simulink model "AerodynamicMoment"  (R2023b)
settings: Solver=VariableStepAuto  StartTime=0.0  StopTime=Tfinal  RelTol=1e-3
model workspace (MAT data in the model file):
  areas = [26.28; 12; 3; 7.5; 17.1; 53.96; 53.96; 4.5; 26.28; 20.1]
  centroids = [4.30109589041  0  1.69726027397; 8.04  1.25  2.4; 7.44  1.25  4.8; 0  1.25  1.5; 3.42  1.25  3; 4.02  9.6  2.3; 4.02  9.6  2.3; 6.84  1.25  3.9; 4.30109589041  0  1.69726027397; 4.02  1.25  0]
  normalVectors = [0  -1  0; 1  0  0; 0  0  1; -1  0  0; 0  0  1; 0  0  1; 0  0  -1; -1  0  0; 0  1  0; 0  0  -1]
  rcm = [4.05894270882 1.95833333333 1.80412649485]
  sequence = "313"
  u0 = [2.10277093747; 1.71391332546; 1.66166340364]
values from neighbouring files (symbols this model uses):
  A_ptob = [0.00452111179393  0.994865050863  -0.101109297888; -0.99864921572  -0.000741813086313  -0.051953764597; -0.0517619888586  0.101207609816  0.993517848971]    [magConstants.mat]
settings Model: Creator=stanforduser  LastModifiedBy=annahylbert
settings DataIOCC: ReturnWorkspaceOutputs=off

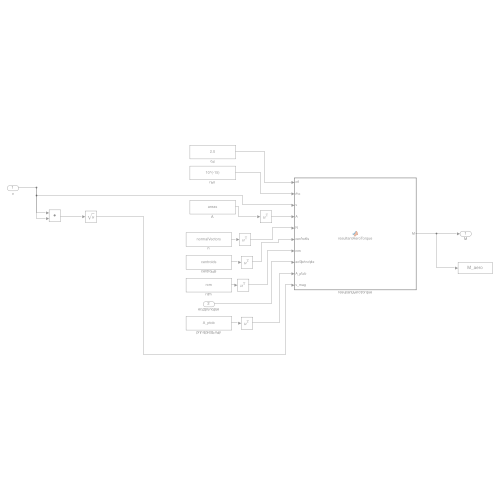
[thumbnail: Simulink's stored preview of the top-level diagram]
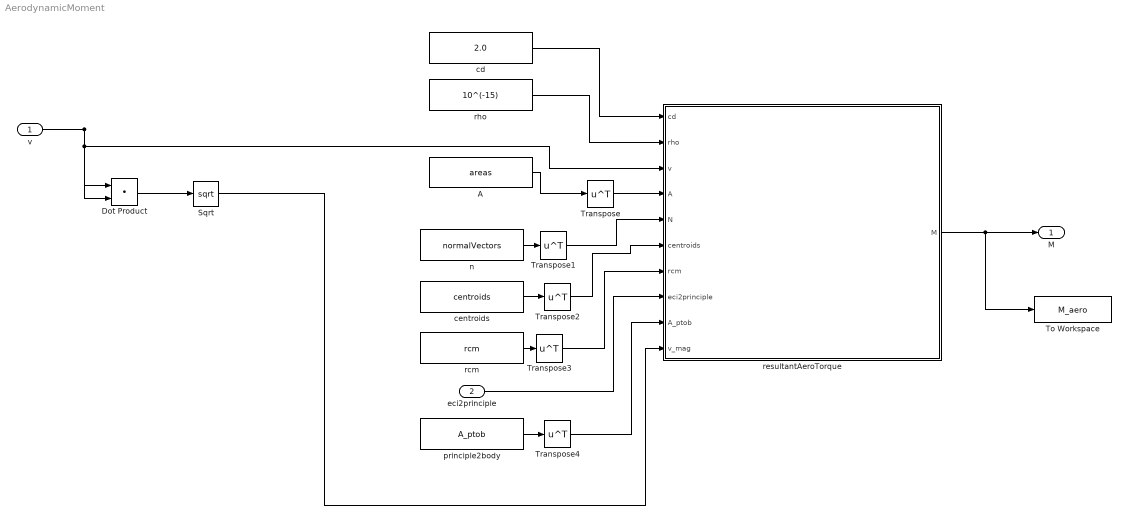
== system AerodynamicMoment ==
  v : Inport  PortDimensions=[3 1]
  eci2principle : Inport  Port=2  PortDimensions=[3 3]
  A : Constant  Value=areas  VectorParams1D=off
  Dot Product : DotProduct  OutDataTypeStr=Inherit: Inherit via internal rule
  Sqrt : Sqrt  OutputSignalType=real
  To Workspace : ToWorkspace  VariableName=M_aero  SampleTime=-1
      settings: Save2DSignal=2-D array (concatenate along first dimension)
  Transpose{,1..4} (5 alike) : Math  Operator=transpose
  cd : Constant  Value=2.0  VectorParams1D=off
  centroids : Constant  Value=centroids  VectorParams1D=off
  n : Constant  Value=normalVectors  VectorParams1D=off
  principle2body : Constant  Value=A_ptob  VectorParams1D=off
  rcm : Constant  Value=rcm  VectorParams1D=off
  resultantAeroTorque : MATLAB Function  TreatAsAtomicUnit=on
  rho : Constant  Value=10^(-15)  VectorParams1D=off
  M : Outport
  wires:
  eci2principle/1 -> resultantAeroTorque/8(eci2principle)
  cd/1 -> resultantAeroTorque/1(cd)
  A/1 -> Transpose/1
  rho/1 -> resultantAeroTorque/2(rho)
  v/1 -> Dot Product/2, resultantAeroTorque/3(v), Dot Product/1
  Dot Product/1 -> Sqrt/1
  Sqrt/1 -> resultantAeroTorque/10(v_mag)
  Transpose/1 -> resultantAeroTorque/4(A)
  centroids/1 -> Transpose2/1
  rcm/1 -> Transpose3/1
  principle2body/1 -> Transpose4/1
  n/1 -> Transpose1/1
  Transpose1/1 -> resultantAeroTorque/5(N)
  Transpose2/1 -> resultantAeroTorque/6(centroids)
  Transpose3/1 -> resultantAeroTorque/7(rcm)
  Transpose4/1 -> resultantAeroTorque/9(A_ptob)
  resultantAeroTorque/1(M) -> To Workspace/1, M/1

== matlab function AerodynamicMoment/resultantAeroTorque ==
  data: cd input; M output; rho input; v input; A input; N input; centroids input; rcm input; eci2principle input; A_ptob input; v_mag input
function M = resultantAeroTorque(cd, rho, v, A, N, centroids, rcm, eci2principle, A_ptob, v_mag)
force = zeros([3 1]);
M = zeros([3 1]);
n = size(A, 1);

%Rotate everything to principle frame
v = eci2principle*v;
rcm = A_ptob * rcm;
for i=1:n
    N(:, i) = A_ptob * N(:, i);
    centroids(:, i) = A_ptob * centroids(:, i);
end 


vUnit = v ./ v_mag;

for i=1:n
    if dot(N(:, i), vUnit) > 0
        force = -0.5 .* cd .* rho .* v_mag^2 .* A(i) .* dot(N(:, i), vUnit) .* vUnit;
        M = M + cross(centroids(:, i) - rcm, force);
    end
end
